simulink model "untitled"  (R2014b)
settings: Solver=ode23s  StartTime=0.0  StopTime=35  RelTol=1e-6
values from neighbouring files (symbols this model uses):
  delta0 = double(delta)    [CalcSteady1.m]    (also in Main2.m)
  J = (1/2)*(H*S)/(ws^2)    (= 7029.15711519)    [CalcSteady1.m]    (also in CalcSteady2.m; Main.m = 3.75; Main2.m = 18500)
  Lq = 5.61e-3    (= 0.00561)    [CalcSteady1.m]    (also in CalcSteady2.m; Main.m; Main2.m; SolverODE.m)
  phi_D0 = double(phi_d)    [CalcSteady1.m]    (also in Main2.m)
  phi_F0 = double(phi_f)    [CalcSteady1.m]    (also in Main2.m)
  phi_Q0 = double(phi_q)    [CalcSteady1.m]    (also in Main2.m)
  Rf = 0.985e-3    (= 0.000985)    [CalcSteady1.m]    (also in CalcSteady2.m; Main.m; Main2.m; SolverODE.m)
  Rs = 1.6e-3    (= 0.0016)    [CalcSteady1.m]    (also in CalcSteady2.m; Main.m; Main2.m; SolverODE.m)
  Tm0 = double(Tm)    [CalcSteady1.m]    (also in Main.m = Tm; Main2.m)
  Vf = Rf*If    [CalcSteady1.m]    (also in CalcSteady2.m; Main.m = double(Rf*If); Main2.m = double(Rf*If); SolverODE.m = Vf0)
  Vrms = 20e3    (= 20000)    [CalcSteady1.m]    (also in Main.m = 22000; Main2.m; SolverODE.m = 22000)
  Wm0 = double(ws)    [CalcSteady1.m]    (also in Main2.m)
settings Model: Creator=Eduardo  LastModifiedBy=Eduardo Montilva

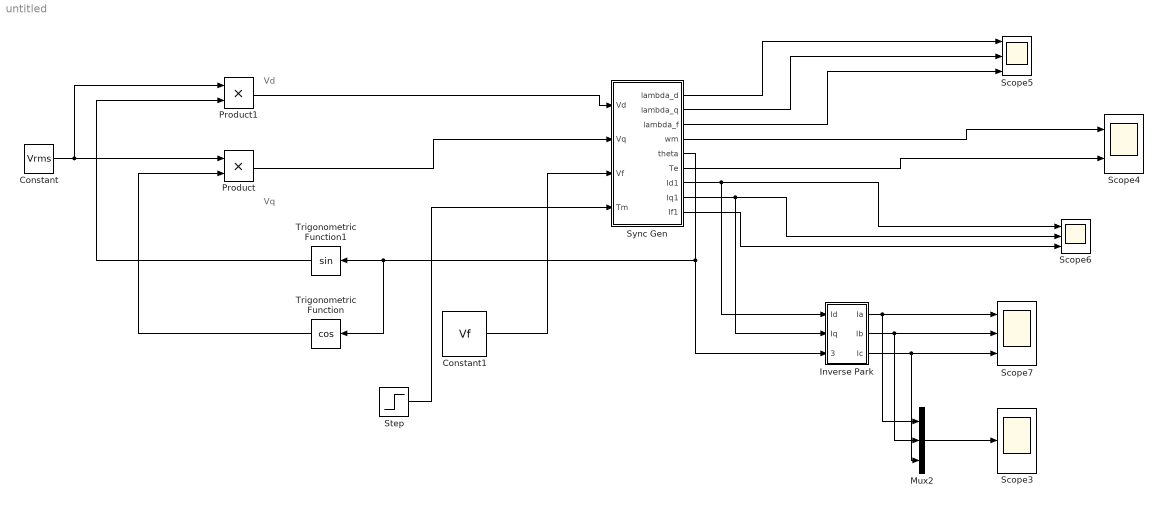
== system untitled ==
  note: Vq
  note: Vd
  Constant : Constant  Value=Vrms
  Constant1 : Constant  Value=Vf
  Inverse Park : Subsystem
  Mux2 : Mux  Inputs=3
  Product : Product
  Product1 : Product
  Scope3 : Scope
      settings: TimeRange=0.001027478145678273  YMin=-3000  YMax=3000
  Scope4 : Scope  NumInputPorts=2
      settings: YMin=0~-5e+06  YMax=1500~5e+06  SaveName=ScopeData4
  Scope5 : Scope  NumInputPorts=3
      settings: YMin=-2000~-40000~-100  YMax=2000~0~100  SaveName=ScopeData5
  Scope6 : Scope  NumInputPorts=3
      settings: YMin=-200000~-10000~-200000  YMax=200000~10000~200000  SaveName=ScopeData6
  Scope7 : Scope  NumInputPorts=3
      settings: TimeRange=0.001027478145678273  YMin=0~0~0  YMax=1~1~1  SaveName=ScopeData7
  Step : Step  Before=Tm0  After=1.2*Tm0  SampleTime=0
  Sync Gen : Subsystem
  Trigonometric Function : Trigonometry  Operator=cos
  Trigonometric Function1 : Trigonometry
  wires:
  Constant1/1 -> Sync Gen/3(Vf)
  Inverse Park/1(Ia) -> Mux2/1, Scope7/1
  Inverse Park/2(Ib) -> Mux2/2, Scope7/2
  Inverse Park/3(Ic) -> Mux2/3, Scope7/3
  Mux2/1 -> Scope3/1
  Step/1 -> Sync Gen/4(Tm)
  Sync Gen/5(theta) -> Inverse Park/3(Theta), Trigonometric Function/1, Trigonometric Function1/1
  Constant/1 -> Product1/1, Product/1
  Trigonometric Function1/1 -> Product1/2
  Trigonometric Function/1 -> Product/2
  Product1/1 -> Sync Gen/1(Vd)
  Product/1 -> Sync Gen/2(Vq)
  Sync Gen/1(lambda_d) -> Scope5/1
  Sync Gen/2(lambda_q) -> Scope5/2
  Sync Gen/3(lambda_f) -> Scope5/3
  Sync Gen/4(wm) -> Scope4/1
  Sync Gen/6(Te) -> Scope4/2
  Sync Gen/7(Id1) -> Inverse Park/1(Id), Scope6/1
  Sync Gen/8(Iq1) -> Inverse Park/2("Iq "), Scope6/2
  Sync Gen/9("If1 ") -> Scope6/3

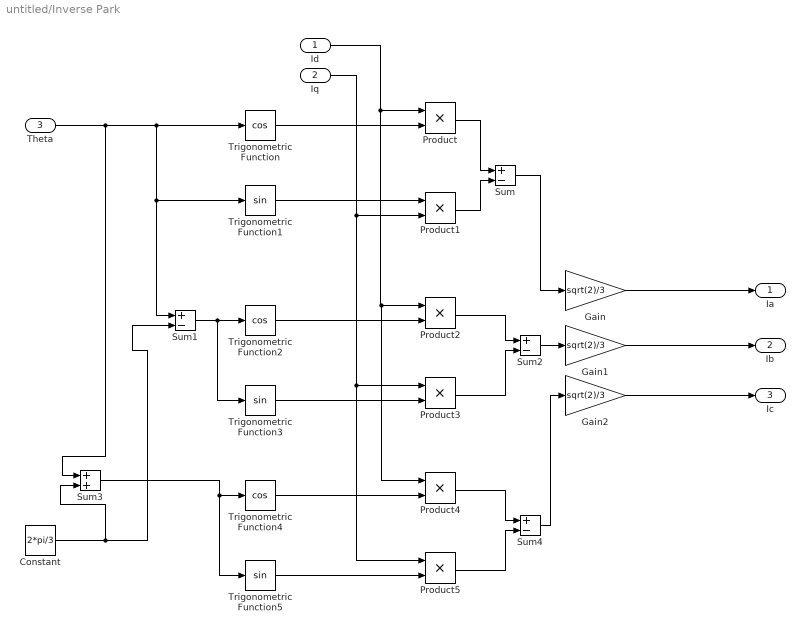
== system untitled/Inverse Park ==
  Id : Inport
  "Iq " : Inport  Port=2
  Theta : Inport  Port=3
  Constant : Constant  Value=2*pi/3
  Gain : Gain  Gain=sqrt(2)/3
  Gain1 : Gain  Gain=sqrt(2)/3
  Gain2 : Gain  Gain=sqrt(2)/3
  Product{,1..5} (6 alike) : Product
  Sum{,1..2,4} (4 alike) : Sum  Inputs=+-
  Sum3 : Sum
  Trigonometric Function : Trigonometry  Operator=cos
  Trigonometric Function1 : Trigonometry
  Trigonometric Function2 : Trigonometry  Operator=cos
  Trigonometric Function3 : Trigonometry
  Trigonometric Function4 : Trigonometry  Operator=cos
  Trigonometric Function5 : Trigonometry
  Ia : Outport
  Ib : Outport  Port=2
  Ic : Outport  Port=3
  wires:
  Gain2/1 -> Ic/1
  Product2/1 -> Sum2/1
  Product3/1 -> Sum2/2
  Sum3/1 -> Trigonometric Function5/1, Trigonometric Function4/1
  Id/1 -> Product/1, Product4/1, Product2/1
  Trigonometric Function4/1 -> Product4/2
  Gain1/1 -> Ib/1
  Sum1/1 -> Trigonometric Function3/1, Trigonometric Function2/1
  Constant/1 -> Sum3/2, Sum1/2
  Sum2/1 -> Gain1/1
  Trigonometric Function2/1 -> Product2/2
  Product/1 -> Sum/1
  Trigonometric Function/1 -> Product/2
  "Iq "/1 -> Product5/1, Product3/1, Product1/2
  Gain/1 -> Ia/1
  Trigonometric Function1/1 -> Product1/1
  Product1/1 -> Sum/2
  Sum/1 -> Gain/1
  Product5/1 -> Sum4/2
  Trigonometric Function5/1 -> Product5/2
  Product4/1 -> Sum4/1
  Sum4/1 -> Gain2/1
  Trigonometric Function3/1 -> Product3/2
  Theta/1 -> Trigonometric Function/1, Trigonometric Function1/1, Sum1/1, Sum3/1

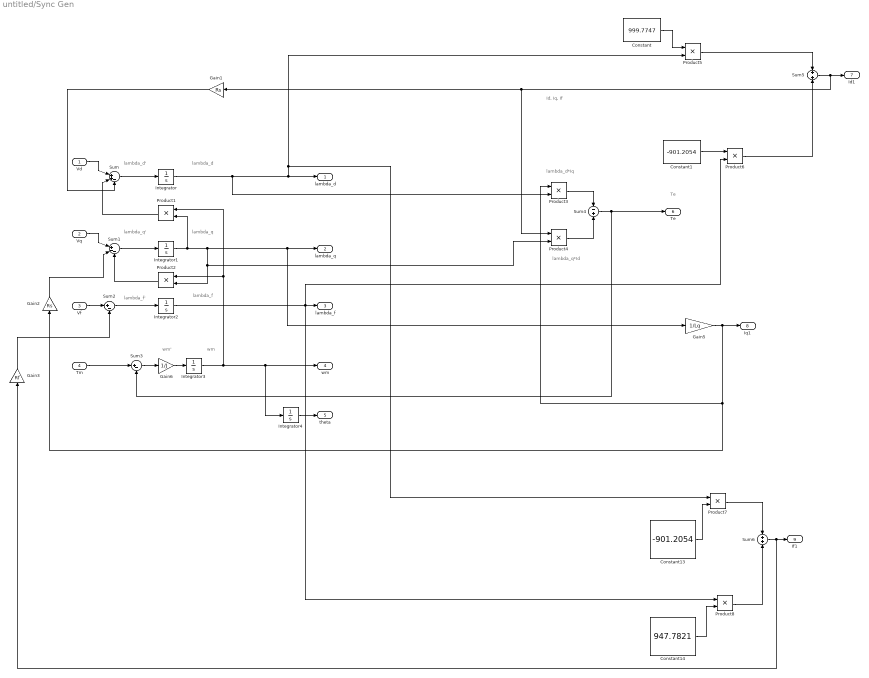
== system untitled/Sync Gen ==
  note: Te
  note: lambda_q*Id
  note: lambda_d*Iq
  note: Id, Iq, If
  note: wm
  note: wm'
  note: lambda_f
  note: lambda_f'
  note: lambda_q
  note: lambda_q'
  note: lambda_d
  note: lambda_d'
  Vd : Inport
  Vq : Inport  Port=2
  Vf : Inport  Port=3
  Tm : Inport  Port=4
  Constant : Constant  Value=999.7747
  Constant1 : Constant  Value=-901.2054
  Constant13 : Constant  Value=-901.2054
  Constant14 : Constant  Value=947.7821
  Gain1 : Gain  Gain=Rs
  Gain2 : Gain  Gain=Rs
  Gain3 : Gain  Gain=Rf
  Gain5 : Gain  Gain=1/Lq
  Gain6 : Gain  Gain=1/J
  Integrator : Integrator  InitialCondition=phi_D0
  Integrator1 : Integrator  InitialCondition=phi_Q0
  Integrator2 : Integrator  InitialCondition=phi_F0
  Integrator3 : Integrator  InitialCondition=Wm0
  Integrator4 : Integrator  InitialCondition=delta0
  Product{1..8} (8 alike) : Product
  Sum : Sum  Inputs=|++-
  Sum1 : Sum  Inputs=|+--
  Sum2 : Sum  Inputs=|+-
  Sum3 : Sum  Inputs=|+-
  Sum4 : Sum  Inputs=-+
  Sum5 : Sum
  Sum6 : Sum
  lambda_d : Outport
  lambda_q : Outport  Port=2
  lambda_f : Outport  Port=3
  wm : Outport  Port=4
  theta : Outport  Port=5
  Te : Outport  Port=6
  Id1 : Outport  Port=7
  Iq1 : Outport  Port=8
  "If1 " : Outport  Port=9
  wires:
  Integrator1/1 -> Product1/2, Product4/2, Product2/2, Gain5/1, lambda_q/1
  Product1/1 -> Sum/2
  Sum2/1 -> Integrator2/1
  Integrator2/1 -> Product8/1, Product6/2, lambda_f/1
  Integrator/1 -> Product7/1, Product5/2, lambda_d/1, Product3/2
  Vq/1 -> Sum1/1
  Sum1/1 -> Integrator1/1
  Vf/1 -> Sum2/1
  Gain1/1 -> Sum/3
  Integrator4/1 -> theta/1
  Gain2/1 -> Sum1/2
  Product2/1 -> Sum1/3
  Gain3/1 -> Sum2/2
  Integrator3/1 -> Product2/1, Product1/1, wm/1, Integrator4/1
  Product3/1 -> Sum4/1
  Product4/1 -> Sum4/2
  Sum/1 -> Integrator/1
  Tm/1 -> Sum3/1
  Vd/1 -> Sum/1
  Sum4/1 -> Sum3/2, Te/1
  Constant/1 -> Product5/1
  Product5/1 -> Sum5/1
  Constant1/1 -> Product6/1
  Product6/1 -> Sum5/2
  Sum5/1 -> Product4/1, Gain1/1, Id1/1
  Gain5/1 -> Product3/1, Gain2/1, Iq1/1
  Gain6/1 -> Integrator3/1
  Sum3/1 -> Gain6/1
  Constant13/1 -> Product7/2
  Constant14/1 -> Product8/2
  Product7/1 -> Sum6/1
  Product8/1 -> Sum6/2
  Sum6/1 -> Gain3/1, "If1 "/1
